simulink model "LUPA"  (R2025b)
settings: Solver=FixedStepAuto  StartTime=0.0  StopTime=inf  FixedStep=Ts  RelTol=1e-3
PreLoadFcn:
  | addpath(genpath('utils'))
model workspace (MAT data in the model file):
  Sig : Simulink.Signal (value not decoded)
values from neighbouring files (symbols this model uses):
  C = 258.803991051052    (= 258.803991051)    [AOE_constants.m]
  CL = 13    [initLUPA.m]
  ExcelGains = table2array(ExcelGains)    [initLUPA.m]
  gainTstep = wavePeriod*10    (= 22.5)    [initLUPA.m]
  Kt = 7.86    [initLUPA.m]
  rampTime = 20    [initLUPA.m]
  sprocketPitchRadius = 0.101854    [initLUPA.m]
  Ts = 0.001    [initLUPA.m]
undefined symbols (not defined in the file or in its folder): AOE, DiscIntNeverNeededParam, drawWire_m, drawWire_mpers, eCATstate, linearPower_W, netForce_N, opState, pos_filt_rad, tet, vel_filt_radpers
libraries: slrealtimeethercatlib x16, slrealtimeloglib x10, simulink x7, dspfdesign x6, eeGeneralControl x3, slrealtimeutilitieslib x2, dspstat3 x2, slrealtimeptplib x1, slrealtimetgmanagement x1
(part 2 of 2)

== matlab function LUPA/CustomControl/Temperature Tank Box Unit1 ==
  data: P input; T output; Rs input; V input; m input
function T = fcn(P,Rs,V,m)

T = P*V/(m*Rs);

== matlab function LUPA/CustomControl/Volume Chamber1 Box Unit1 ==
  data: x input; A input; V output; L input
% function V = fcn(x,A,L)
% V = A*(-x +L);

function V = fcn(x,A,L)

if L - x < 0.05*L
    V = A*(0.05*L);
else
    V = A*(-x +L);
end

== matlab function LUPA/CustomControl/Revised Cylinder Outlet Valve Model ==
  data: mdotMaxOld input; TimeStep input; PC input; TC input; xdot input; x input; LC input; AC input; DC input; Rs input; gma input; Tw input; hC input; MassFlow output; hT input; aT input; VT input; PT input; TT input; A input; mdotMax output; beta output
function [MassFlow, mdotMax, beta]   = fcn(mdotMaxOld, TimeStep, PC, TC,xdot ,x, LC,AC, DC,Rs,gma,Tw,hC, hT, aT, VT, PT, TT, A)

if PC >= PT
    beta = PT/PC;
    
    if beta > 0.999
        beta = 0.999;
    end
    
    if beta > 0.5283
        mdotMax = A*PC*sqrt(abs((2*gma/((gma-1)*Rs*TC))*((beta)^(2/gma) - (beta)^((gma+1)/gma)))); %subsonic
    else
        mdotMax = 0.0404*PC*A/sqrt(TC); %sonic
    end
    
else
    mdotMax = 0;
    beta = 0;
end

%Calculating Volumes/Areas
% VC = AC*(x +LC);
% aC = pi*DC*(x +LC) + 2*AC; %heat transfer area
if LC+x < 0.05*LC
    VC = AC*(0.05*LC);
    aC = pi*DC*(0.05*LC) + 2*AC; %heat transfer area
else
    VC = AC * (x +LC);
    aC = pi*DC*(x +LC) + 2*AC; %heat transfer area
end

if TimeStep == 0
    MassFlow = 0;
    %MassFlow_Opt = 0;
    %MassFlow_Opt2 = 0;
    PdotC = 0;
    Change = 0;
else
    Change = 0;
    
    
%     %Determining what the tank properties will be in the next time step
%     
%     PT = PT + Pdot*TimeStep;
%     TT = PT*VT/(Tmass*Rs);
%     
%     %Determining what the cylinder properties will be in the next time step
%     PdotC = (-1*gma*PC*(xdot)*AC - (gma-1)*hC*aC*(TC-Tw) - gma*Rs*TC*MassFlowOld)/VC;
%     PC = PC + PdotC*TimeStep;
%     TC = PC*VC/(Cmass*Rs);
    
    %Determining what the pressure needs to be in the following time step
    %P2 = (TimeStep/(VT+VC))*( (PT*VT/TimeStep) + (PC*VC/TimeStep) - gma*PC*(xdot)*AC - (gma-1)*hC*aC*(TC-Tw) -(gma-1)*hT*aT*(TT-Tw) + gma*Rs*TT*mDotT);
    P2 = (TimeStep/(VT+VC))*( (PT*VT/TimeStep) + (PC*VC/TimeStep) - gma*PC*(xdot)*AC - (gma-1)*hC*aC*(TC-Tw) -(gma-1)*hT*aT*(TT-Tw));
    
    MassFlow_Opt = (1/(Rs*TC*gma))*( -(P2 - PC)*VC/TimeStep - gma*PC*(xdot)*AC - (gma-1)*hC*aC*(TC-Tw) );
    %MassFlow_Opt2 = (1/(Rs*TC*gma))*( (P2 - PT)*VT/TimeStep + (gma-1)*hT*aT*(TT-Tw) - gma*Rs*TT*mDotT);
    
    MassFlow = MassFlow_Opt*0.99;
    
    PdotC = (-1*gma*PC*(xdot)*AC - (gma-1)*hC*aC*(TC-Tw) - gma*Rs*TC*MassFlow )/VC;
end

if MassFlow < 0
    MassFlow = 0;
end

if MassFlow > mdotMax
    if mdotMaxOld > mdotMax
        if MassFlow > mdotMaxOld
            MassFlow = mdotMaxOld;
        end
        mdotMax = mdotMaxOld;
    else
        MassFlow = mdotMax;
    end
end

% if Change == 1
%     PdotC = (-1*gma*PC*(xdot)*AC - (gma-1)*hC*aC*(TC-Tw) - gma*Rs*TC*MassFlow )/VC;
% end

PCPredicted = PC + PdotC*TimeStep;

== matlab function LUPA/CustomControl/Revised Valve Tank Outlet ==
  data: mdotMaxOld input; TimeStep input; PT input; TT input; Rs input; gma input; Tw input; hT input; VT input; aT input; MassFlow output; Pcrack input; TC input; mDotIn input; A input; mdotMax output; beta output
function [MassFlow, mdotMax, beta]   = fcn(mdotMaxOld, TimeStep, PT, TT ,Rs,gma,Tw,hT, VT, aT, Pcrack, TC, mDotIn, A)

%Determine Maximum Mass Flow Rate

%A is orifice area

if PT >= Pcrack
    beta = Pcrack/PT;
    
    %This prevents instabilities as Beta approaches 1
    if beta > 0.999
        beta = 0.999;
    end
    
    if beta > 0.5283
        mdotMax = A*PT*sqrt(abs((2*gma/((gma-1)*Rs*TT))*((beta)^(2/gma) - (beta)^((gma+1)/gma)))); %subsonic
    else
        mdotMax = 0.0404*PT*A/sqrt(TT); %sonic
    end
    
else
    mdotMax = 0;
    beta = 0;
end

if TimeStep == 0
    MassFlow = 0;
else
    %Determining what the pressure needs to be in the following time step
    P2 = Pcrack;
    
    MassFlow_Opt = (1/(Rs*TT*gma))*( -(P2 - PT)*VT/TimeStep - (gma-1)*hT*aT*(TT-Tw) + gma*Rs*TC*mDotIn);
    
    MassFlow = MassFlow_Opt*0.99;
end

if MassFlow < 0
    MassFlow = 0;
end

if MassFlow > mdotMax
    if mdotMaxOld > mdotMax
        if MassFlow > mdotMaxOld
            MassFlow = mdotMaxOld;
        end
        mdotMax = mdotMaxOld;
    else
        MassFlow = mdotMax;
    end
end
    
end

== matlab function LUPA/CustomControl/Revised Valve Model Inlet Unit1 ==
  data: mdotMaxOld input; TimeStep input; PC1 input; TC1 input; xdot input; x input; LC input; AC input; DC input; Rs input; gma input; Tw input; hC input; Tamb input; A input; MassFlow output; Pin input; mdotMax output
function [MassFlow, mdotMax]   = fcn(mdotMaxOld, TimeStep, PC1, TC1,xdot ,x, LC,AC, DC,Rs,gma,Tw,hC, Tamb, A, Pin)

if Pin >= PC1
    beta = PC1/Pin;
    
    if beta > 0.999
        beta = 0.999;
    end
    
    if beta > 0.5283
        mdotMax = A*Pin*sqrt(abs((2*gma/((gma-1)*Rs*Tamb))*((beta)^(2/gma) - (beta)^((gma+1)/gma)))); %subsonic
    else
        mdotMax = 0.0404*Pin*A/sqrt(Tamb); %sonic
    end
    
else
    mdotMax = 0;
end

if TimeStep == 0
    MassFlow = 0;
else
    %Calculating Volumes/Areas
    % VC = AC*(-x +LC);
    % aC = pi*DC*(-x +LC) + 2*AC; %heat transfer area
    if LC - x < 0.05*LC
        VC = AC*(0.05*LC);
        aC = pi*DC*(0.05*LC) + 2*AC; %heat transfer area
    else
        VC = AC*(-x +LC);
        aC = pi*DC*(-x +LC) + 2*AC;
    end
    
    %Determining what the pressure needs to be in the following time step
    P2 = Pin;
    
    MassFlow_Opt = (1/(Rs*Tamb*gma))*( (P2 - PC1)*VC/TimeStep + gma*PC1*(-xdot)*AC + (gma-1)*hC*aC*(TC1-Tw) );
    MassFlow = MassFlow_Opt*0.99;

end

if MassFlow < 0
    MassFlow = 0;
end

if MassFlow > mdotMax
    if mdotMaxOld > mdotMax
        if MassFlow > mdotMaxOld
            MassFlow = mdotMaxOld;
        end
        mdotMax = mdotMaxOld;
    else
        MassFlow = mdotMax;
    end
end

== matlab function LUPA/CustomControl/Revised Valve Model Chamber1Chamber2 Unit1 ==
  data: mdotMaxOld input; TimeStep input; xdot input; x input; PC1 input; TC1 input; LC input; AC input; DC input; Rs input; gma input; Tw input; hC input; MassFlow output; PC2 input; TC2 input; A input; mdotMax output
function [MassFlow, mdotMax]   = fcn(mdotMaxOld, TimeStep, xdot ,x,PC1, TC1, LC,AC, DC,Rs,gma,Tw,hC, PC2, TC2, A)

if PC1 >= PC2
    beta = PC2/PC1;
    
    if beta > 0.999
        beta = 0.999;
    end
    
    if beta > 0.5283
        mdotMax = A*PC1*sqrt(abs((2*gma/((gma-1)*Rs*TC1))*((beta)^(2/gma) - (beta)^((gma+1)/gma)))); %subsonic
    else
        mdotMax = 0.0404*PC1*A/sqrt(TC1); %sonic
    end
    
else
    mdotMax = 0;
end

if TimeStep == 0
    MassFlow = 0;
else
    % %Calculating Volumes/Areas
    % VC1 = AC*(-x +LC);
    % aC1 = pi*DC*(-x +LC) + 2*AC; %heat transfer area
    if LC - x < 0.05*LC
        VC1 = AC*(0.05*LC);
        aC1 = pi*DC*(0.05*LC) + 2*AC; %heat transfer area
    else
        VC1 = AC*(-x +LC);
        aC1 = pi*DC*(-x +LC) + 2*AC;
    end

    % VC2 = AC*(x +LC);
    % aC2 = pi*DC*(x +LC) + 2*AC; %heat transfer area
    if LC+x < 0.05*LC
        VC2 = AC*(0.05*LC);
        aC2 = pi*DC*(0.05*LC) + 2*AC; %heat transfer area
    else
        VC2 = AC * (x +LC);
        aC2 = pi*DC*(x +LC) + 2*AC; %heat transfer area
    end
    
    %Determining what the pressure needs to be in the following time step
    P2 = (TimeStep/(VC2+VC1))*( (PC2*VC2/TimeStep) + (PC1*VC1/TimeStep) - gma*PC1*(-xdot)*AC - (gma-1)*hC*aC1*(TC1-Tw) - gma*PC2*xdot*AC - (gma-1)*hC*aC2*(TC2-Tw));

    MassFlow_Opt = (1/(Rs*TC1*gma))*( -(P2 - PC1)*VC1/TimeStep - gma*PC1*(-xdot)*AC - (gma-1)*hC*aC1*(TC1-Tw) );
    MassFlow = MassFlow_Opt*0.99;

end

if MassFlow < 0
    MassFlow = 0;
end

if MassFlow > mdotMax
    if mdotMaxOld > mdotMax
        if MassFlow > mdotMaxOld
            MassFlow = mdotMaxOld;
        end
        mdotMax = mdotMaxOld;
    else
        MassFlow = mdotMax;
    end
end

== matlab function LUPA/CustomControl/Volume Chamber2 Box Unit1 ==
  data: x input; A input; V output; L input
% function V = fcn(x,A,L)
% 
% V = A*(x +L);

function V = fcn(x,A,L)

if L+x < 0.05*L
    V = A*(0.05*L);
else
    V = A*(x +L);

end

== matlab function LUPA/CustomControl/Pressure Chamber1 Box Unit1 ==
  data: P input; T input; xdot input; x input; Tin1 input; mdot1 input; mdot3 input; L input; A input; D input; Rs input; gma input; Tw input; h input; Pdot output
function Pdot = fcn(P, T,xdot ,x, Tin1, mdot1,mdot3,L,A, D,Rs,gma,Tw,h)

% V = A*(-x +L);
% a = pi*D*(-x +L) + 2*A; %heat transfer area

if L - x < 0.05*L
    V = A*(0.05*L);
    a = pi*D*(0.05*L) + 2*A; %heat transfer area
else
    V = A*(-x +L);
    a = pi*D*(-x +L) + 2*A; %heat transfer area
end

Pdot = (-1*gma*P*(-xdot)*A - (gma-1)*h*a*(T-Tw) + gma*Rs*Tin1*mdot1 - gma*Rs*T*mdot3)/V;

== matlab function LUPA/CustomControl/Pressure Tank Box Unit1 ==
  data: T input; Tin input; mdot1 input; mdot2 input; Rs input; gma input; h input; a input; V input; Tw input; Pdot output
function Pdot  = fcn(T, Tin, mdot1,mdot2,Rs,gma,h, a, V,Tw)

Pdot = (-(gma-1)*h*a*(T-Tw) + gma*Rs*Tin*mdot1 - gma*Rs*T*mdot2)/V;

== matlab function LUPA/Control/MATLAB Function ==
  data: controllerType input; x input; I_ctrl output; manualGains input; stiffness_Nperm output; time input; GainTstep input; ExcelGains input; Kt input; sprocketPitchRadius input; damping_Npermpers output
function [I_ctrl, stiffness_Nperm, damping_Npermpers] = fcn(controllerType, x, manualGains,time,GainTstep,ExcelGains, Kt, sprocketPitchRadius)
% gain format [positionProportional, velocityProportional]
% x format [theta; omega]

I_ctrl = 0;
gainMat = zeros(1,2);

if controllerType == 1

    B = sprocketPitchRadius^2 / Kt * manualGains' * x;
    stiffness_Nperm = manualGains(1);
    damping_Npermpers = manualGains(2);
elseif controllerType == 2
    idx = ceil(time./GainTstep); % Find index of current gain step
    while idx > length(ExcelGains(:,1))
        idx = idx-length(ExcelGains(:,1));
    end
    gainMat(1,1) = ExcelGains(idx,1);
    gainMat(1,2) = ExcelGains(idx,2);
    B = sprocketPitchRadius^2 / Kt * gainMat* x;
    stiffness_Nperm = gainMat(1,1);
    damping_Npermpers = gainMat(1,2);
else
    B = 0;
    stiffness_Nperm = 0;
    damping_Npermpers = 0;
end

I_ctrl = B;

== matlab function LUPA/Initialization/controlword ==
  data: enabled input; clearfault input; statusword input; controlword output
function controlword = fcn(enabled, clearfault, statusword)

bitstatus = bitget(statusword,1:16);

if ~clearfault
    if enabled
        if bitstatus(1) == 0 % Ready to switch on not ready
            controlword = 6; % command ready switch on
        elseif ~bitstatus(2) % switched not yet on
            controlword = 7; % command switch on
        elseif ~bitstatus(3) % operation not yet enabled
            controlword = 15; % command enable
        else
            controlword = 15; % maintain enabled state
        end
    else
        controlword = 4; % command disabled
    end
else
    controlword = 128; % command clear faults
end

== matlab function LUPA/CustomControl/Determining Useful Energy ==
  data: T input; P input; mDot input; Density input; Cp input; Rs input; Tamb input; Pamb input; Exergy output; Power output
function [Exergy, Power]   = fcn(T, P, mDot, Density, Cp, Rs, Tamb, Pamb)
    
%Determining Flow Exergy
Flow_Exergy = Cp*Tamb*( (T/Tamb) - 1 - log(T/Tamb) ) + Rs*Tamb*log(P/Pamb);

Exergy = Flow_Exergy*mDot; %This has the units of Watts

%Determining Energy of Output
Power = mDot*(P - Pamb)/Density;

end

== matlab function LUPA/CustomControl/Pressure Chamber2 Box Unit1 ==
  data: P input; T input; xdot input; x input; Tin1 input; mdot1 input; mdot3 input; L input; A input; D input; Pdot output; Rs input; gma input; Tw input; h input
function Pdot = fcn(P, T,xdot ,x, Tin1, mdot1,mdot3,L,A, D,Rs,gma,Tw,h)

% V = A * (x +L);
% a = pi*D*(x +L) + 2*A; %heat transfer area

if L+x < 0.05*L
    V = A*(0.05*L);
    a = pi*D*(0.05*L) + 2*A; %heat transfer area
else
    V = A * (x +L);
    a = pi*D*(x +L) + 2*A; %heat transfer area
end

Pdot = (-1*gma*P*(xdot)*A - (gma-1)*h*a*(T-Tw) + gma*Rs*Tin1*mdot1 - gma*Rs*T*mdot3)/V;
